simulink model "FFR_1_0"  (R2015a)
settings: Solver=ode45  StartTime=0.0  StopTime=15  RelTol=1e-3
values from neighbouring files (symbols this model uses):
  D = 0.015    [init_FFR_1_0.m]    (also in init_FFR_1_1.m; init_FFR_3area.m = [0.015 0.016 0.015]; init_FFR_3area_2.m = [0.015 0.016 0.015]; init_FFR_3area_3.m = [0.015 0.016 0.015])
  H = 0.0833    [init_FFR_1_0.m]    (also in init_FFR_1_1.m; init_FFR_3area.m = [0.1667 0.2017 0.1247] .* 0.5; init_FFR_3area_2.m = [0.1667 0.2017 0.1247] .* 0.5; init_FFR_3area_3.m = [0.1667 0.2017 0.1247] .* 0.5)
  Ki = -0.3    [init_FFR_1_0.m]    (also in init_FFR_1_1.m = -2; init_FFR_3area.m = [-0.3 -0.2 -0.4]; init_FFR_3area_2.m = [-0.3 -0.2 -0.4]; init_FFR_3area_3.m = [-0.3 -0.2 -0.4])
  R = 3    [init_FFR_1_0.m]    (also in init_FFR_1_1.m; init_FFR_3area.m = [3 2.73 2.82]; init_FFR_3area_2.m = [3 2.73 2.82]; init_FFR_3area_3.m = [3 2.73 2.82])
  T_g = 0.08    [init_FFR_1_0.m]    (also in init_FFR_1_1.m; init_FFR_3area.m = [0.08 0.06 0.07]; init_FFR_3area_2.m = [0.08 0.06 0.07]; init_FFR_3area_3.m = [0.08 0.06 0.07])
  T_t = 0.40    (= 0.4)    [init_FFR_1_0.m]    (also in init_FFR_1_1.m; init_FFR_3area.m = [0.40 0.44 0.30]; init_FFR_3area_2.m = [0.40 0.44 0.30]; init_FFR_3area_3.m = [0.40 0.44 0.30])
settings Model: Creator=tarje  LastModifiedBy=tarje

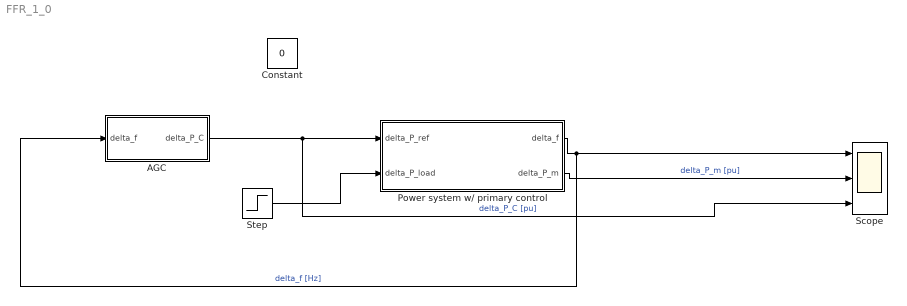
== system FFR_1_0 ==
  AGC : Subsystem
  Constant : Constant  Value=0
  Power system w/ primary control : Subsystem
  Scope : Scope  NumInputPorts=3
      settings: TimeRange=15  YMin=-0.08~-0.005~-0.01  YMax=0.025~0.04~0.03
  Step : Step  Time=2  After=.02  SampleTime=0
  wires:
  Step/1 -> Power system w/ primary control/2(delta_P_load)
  Power system w/ primary control/1(delta_f) -> AGC/1(delta_f), Scope/1  "delta_f [Hz]"
  Power system w/ primary control/2(delta_P_m) -> Scope/2  "delta_P_m [pu]"
  AGC/1(delta_P_C) -> Scope/3, Power system w/ primary control/1(delta_P_ref)  "delta_P_C [pu]"

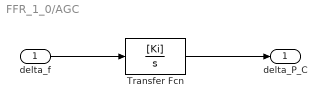
== system FFR_1_0/AGC ==
  delta_f : Inport
  Transfer Fcn : TransferFcn  Numerator=[Ki]  Denominator=[1 0]
  delta_P_C : Outport
  wires:
  delta_f/1 -> Transfer Fcn/1
  Transfer Fcn/1 -> delta_P_C/1

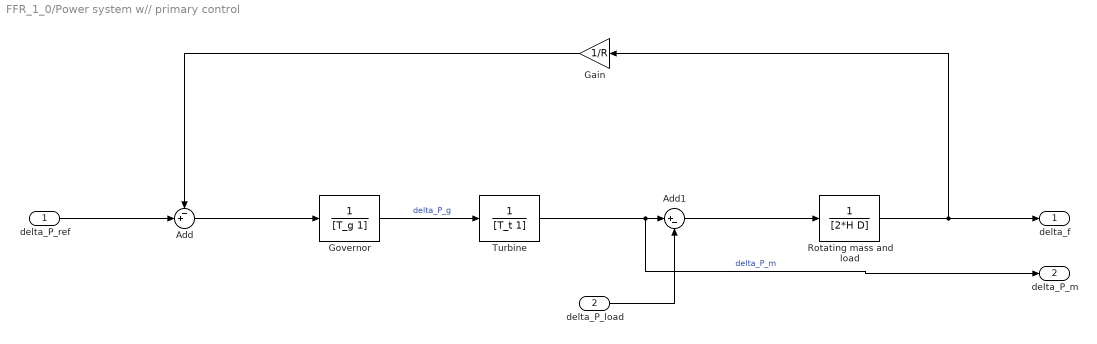
== system FFR_1_0/Power system w// primary control ==
  delta_P_ref : Inport
  delta_P_load : Inport  Port=2
  Add : Sum  Inputs=-+|
  Add1 : Sum  Inputs=|+-
  Gain : Gain  Gain=1/R
  Governor : TransferFcn  Denominator=[T_g 1]
  Rotating mass and load : TransferFcn  Denominator=[2*H D]
  Turbine : TransferFcn  Denominator=[T_t 1]
  delta_f : Outport
  delta_P_m : Outport  Port=2
  wires:
  Turbine/1 -> delta_P_m/1, Add1/1  "delta_P_m"
  Rotating mass and load/1 -> delta_f/1, Gain/1
  Gain/1 -> Add/1
  delta_P_load/1 -> Add1/2
  Add1/1 -> Rotating mass and load/1
  Add/1 -> Governor/1
  Governor/1 -> Turbine/1  "delta_P_g"
  delta_P_ref/1 -> Add/2
